simulink model "pwmController"  (R2018b)
settings: Solver=ode23s  StartTime=0.0  StopTime=0.01  FixedStep=1e-6  RelTol=1e-3
libraries: simulink x2, powerlib_meascontrol x1, powerlib x1
settings Model: Creator=K2  LastModifiedBy=K2

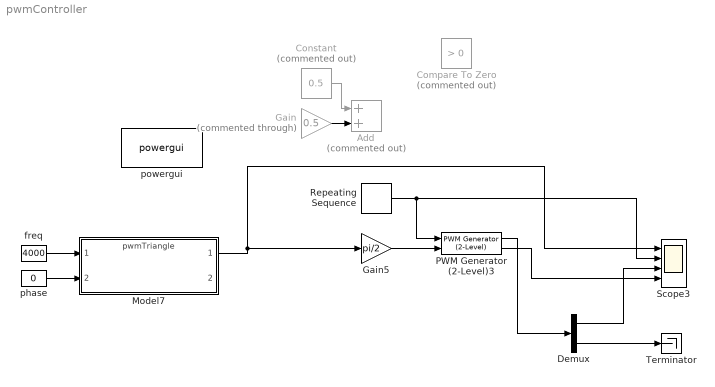
== system pwmController ==
  Add : Sum  Commented=on
  Compare To Zero : simulink/Logic and Bit Operations/Compare To Zero  Commented=on  relop=>  OutDataTypeStr=boolean
  Constant : Constant  Commented=on  Value=0.5
  Demux : Demux  Outputs=2
  Gain : Gain  Commented=through  Gain=0.5
  Gain5 : Gain  Gain=pi/2
  Model7 : ModelReference  ModelNameDialog=pwmTriangle.slx  SimulationMode=Normal  ModelReferenceVersion=1.5
  PWM Generator (2-Level)3 : powerlib_meascontrol/Pulse & Signal Generators/PWM Generator (2-Level)  ModulatorType=Single-phase half-bridge (2 pulses)  ModulatorMode=Synchronized  Fc=freq  Pc=0  nF=1  MinMax=[0.01 1]  SamplingTechnique=Natural  ModulatingSignals=off  m=0.8  Freq=60  Phase=0  Ts=-1  ShowCarrierOutport=on
      settings: SourceProductName=Simscape Power Systems
  Repeating Sequence : simulink/Sources/Repeating Sequence  rep_seq_t="[0 0.001 0.005 0.006   0.0101]"  rep_seq_y=[1 1 0 0 -1]
  Scope3 : Scope  NumInputPorts=4
  Terminator : Terminator
  freq : Constant  Value=4000
  phase : Constant  Value=0
  powergui : powerlib/powergui  Priority=1  SimulationMode=Discrete  SampleTime=1e-6  frequency=60  Iterations=50  frequencyindice=0  Pbase=100e6  ErrMax=1e-4  UnitsV=kV  UnitsW=MW  buscounter=0  FunctionMessages=off  echomessages=off  EnableUseOfTLC=off  CurrentSourceSwitches=off  DisableSnubberDevices=off  DisableRonSwitches=off  DisableVfSwitches=off  DisplayEquations=off  SolverType=Tustin  Interpol=off  ExternalGateDelay=off  methode=off  Ts=100  x0status=blocks  SPID=off  SwTol=0  HookPort=off  RestoreLinks=warning  ResistiveCurrentMeasurement=off  Frange=[0:2:500]  Ylog=off  Xlog=on  ShowGrid=off  save=off  variable=ZData  structure=0  ZoomFFT=off  StartTime=0.0  cycles=1  DisplayStyle=1  fundamental=60  FreqAxis=off  MaxFrequency=1000  frequencyindicesteady=1  RmsSteady=1  display=off
  wires:
  freq/1 -> Model7/1
  phase/1 -> Model7/2
  PWM Generator (2-Level)3/1 -> Demux/1
  Demux/1 -> Scope3/3
  Demux/2 -> Terminator/1
  Gain5/1 -> PWM Generator (2-Level)3/2
  Repeating Sequence/1 -> PWM Generator (2-Level)3/1, Scope3/2
  Model7/1 -> Gain5/1, Scope3/1
  Gain/1 -> Add/2
  Constant/1 -> Add/1
  PWM Generator (2-Level)3/2 -> Scope3/4
